simulink model "test_lift_discretization"  (R2021b)
settings: Solver=VariableStepAuto  StartTime=0.0  StopTime=200  MaxStep=1e-3  RelTol=1e-3
values from neighbouring files (symbols this model uses):
  g = 9.806    [plot_bode_diagram.m]    (also in test_LiftDynamicsEquation.m; test_discretization.m)
  Ts = 1e-3    (= 0.001)    [test_LiftDynamicsEquation.m]    (also in test_discretization.m; test_motion_law.m = 0.01)
  u_eq = Rp.*gearbox.*(dc-dw+Mc.*g-Mw.*g+BuildingHeight.*g.*mu-Rp.*g.*gearbox.*mu.*state9.*2.0)    [LiftEquilibrium.m]    (also in SymbolicEquation.m = simplify(u_eq))
  u_test = 0.99*u_eq    [test_discretization.m]
libraries: LumpedParameterLiftModels x4
settings Model: Creator=manue  LastModifiedBy=manue

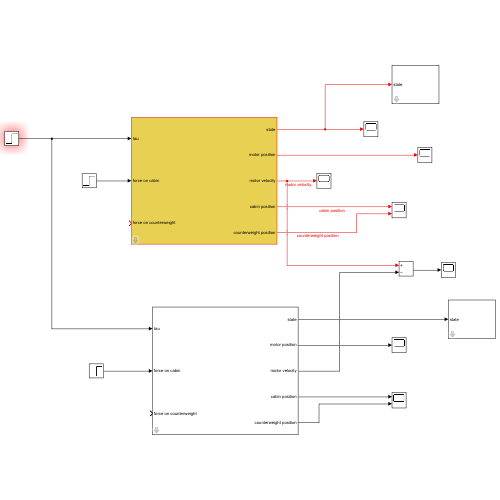
[thumbnail: Simulink's stored preview of the top-level diagram]
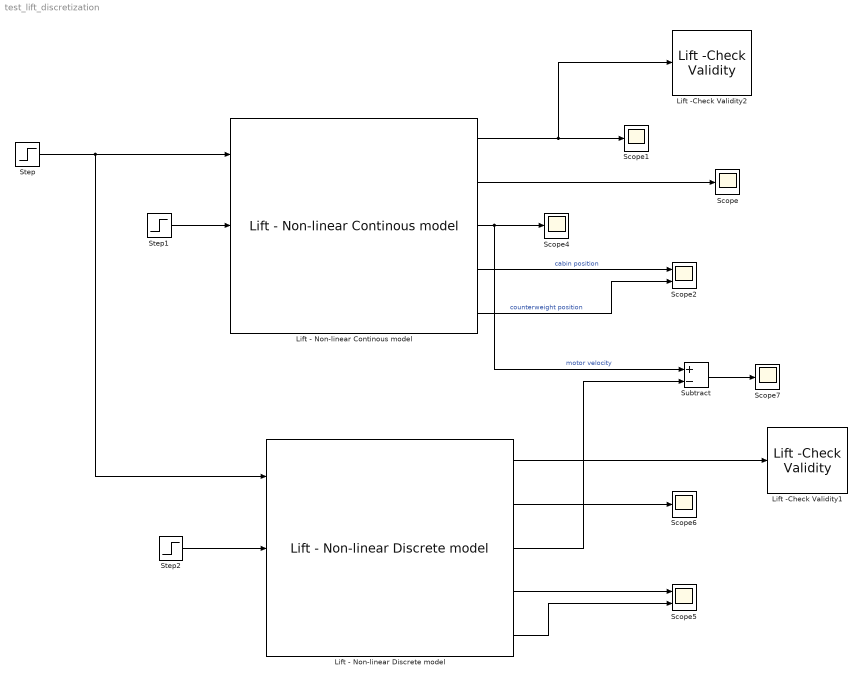
== system test_lift_discretization ==
  Lift - Non-linear Continous model : LumpedParameterLiftModels/Lift - Non-linear Continous model  Jp=Jp  Jm=Jm  Mc=Mc  Mw=Mw  LinearStiffness=LinearStiffness  LinearDamping=LinearDamping  Rp=Rp  mu=mu  BuildingHeight=BuildingHeight  MotorViscousFriction=MotorViscousFriction  g=g  gearbox=gearbox  min_length=min_length  x9_init=0
  Lift - Non-linear Discrete model : LumpedParameterLiftModels/Lift - Non-linear Discrete model  Jp=Jp  Jm=Jm  Mc=Mc  Mw=Mw  LinearStiffness=LinearStiffness  LinearDamping=LinearDamping  Rp=Rp  mu=mu  BuildingHeight=BuildingHeight  MotorViscousFriction=MotorViscousFriction  g=g  gearbox=gearbox  min_length=min_length  x9_init=0  Ts=Ts
  Lift -Check Validity1 : LumpedParameterLiftModels/Lift -Check Validity  BuildingHeight=BuildingHeight  min_length=min_length
  Lift -Check Validity2 : LumpedParameterLiftModels/Lift -Check Validity  BuildingHeight=BuildingHeight  min_length=min_length
  Scope{,1,4,6..7} (5 alike) : Scope
  Scope2 : Scope  NumInputPorts=2
  Scope5 : Scope  NumInputPorts=2
  Step : Step  Time=100  Before=u_eq  After=u_test  SampleTime=0
  Step1 : Step  Time=20  After=0  SampleTime=0
  Step2 : Step  Time=20  After=0  SampleTime=0
  Subtract : Sum  Inputs=+-
  wires:
  Lift - Non-linear Continous model/2 -> Scope/1
  Lift - Non-linear Continous model/1 -> Lift -Check Validity2/1, Scope1/1
  Lift - Non-linear Continous model/4 -> Scope2/1  "cabin position"
  Lift - Non-linear Continous model/5 -> Scope2/2  "counterweight position"
  Step1/1 -> Lift - Non-linear Continous model/2
  Lift - Non-linear Continous model/3 -> Scope4/1, Subtract/1  "motor velocity"
  Lift - Non-linear Discrete model/3 -> Subtract/2
  Lift - Non-linear Discrete model/4 -> Scope5/1
  Lift - Non-linear Discrete model/5 -> Scope5/2
  Lift - Non-linear Discrete model/2 -> Scope6/1
  Subtract/1 -> Scope7/1
  Step2/1 -> Lift - Non-linear Discrete model/2
  Step/1 -> Lift - Non-linear Discrete model/1, Lift - Non-linear Continous model/1
  Lift - Non-linear Discrete model/1 -> Lift -Check Validity1/1
